simulink model "ES005A_TmplMonr"  (R2013b)
settings: Solver=FixedStepDiscrete  SolverMode=SingleTasking  StartTime=0.0  StopTime=1  FixedStep=0.002  RelTol=1e-3
undefined symbols (not defined in the file): ELECGLBPRM_STRTUPSTDI_CNT_U08, ELECGLBPRM_STRTUPSTTMPLMONININTESTSTRT_CNT_U08, IninFlt, RtFlt, SpiConf_SpiChannel_TmplMonrCh1, SpiConf_SpiChannel_TmplMonrCh2, SpiConf_SpiChannel_TmplMonrCh3, SpiConf_SpiSequence_TmplMonrSeq1, SpiConf_SpiSequence_TmplMonrSeq2, SpiConf_SpiSequence_TmplMonrSeq3, STD_HIGH, STD_LOW, TMPLMONRCFGREG1READVAL_CNT_U16, TMPLMONRCFGREG1WRVAL_CNT_U16, TMPLMONRSTSREG2READVAL_CNT_U16, TMPLMONRWDGMODKEYWORD1_CNT_U16, TMPLMONRWDGMODKEYWORD2_CNT_U16, TMPLMONRWDGMODKEYWORD3_CNT_U16, TrigReg1
libraries: simulink x12
(part 1 of 4)
settings Model: Creator=HZY4G9  LastModifiedBy=fz41t8
settings SolverCC: AutoInsertRateTranBlk=on  InsertRTBMode=Always
settings DataIOCC: LimitDataPoints=off  SaveFormat=Structure  ReturnWorkspaceOutputs=on
settings OptimizationCC: BlockReduction=off  InlineParams=on  ZeroExternalMemoryAtStartup=off  ZeroInternalMemoryAtStartup=off  OptimizeModelRefInitCode=on  LifeSpan=1
settings DebuggingCC: SignalInfNanChecking=error  SignalRangeChecking=warning  UnderspecifiedInitializationDetection=Simplified  SolverPrmCheckMsg=error  InheritedTsInSrcMsg=error  DiscreteInheritContinuousMsg=error  SingleTaskRateTransMsg=error  TasksWithSamePriorityMsg=error  SigSpecEnsureSampleTimeMsg=error  CheckMatrixSingularityMsg=error  ParameterUnderflowMsg=error  ParameterPrecisionLossMsg=error  ParameterTunabilityLossMsg=error  FixptConstUnderflowMsg=warning  FixptConstOverflowMsg=warning  VectorMatrixConversionMsg=error  SignalLabelMismatchMsg=error  UnconnectedInputMsg=error  UnconnectedOutputMsg=error  UnconnectedLineMsg=error  SFcnCompatibilityMsg=error  UniqueDataStoreMsg=warning  BusObjectLabelMismatch=error  RootOutportRequireBusObject=error  AssertControl=DisableAll  ModelReferenceIOMsg=error  ModelReferenceVersionMismatchMessage=warning  ModelReferenceIOMismatchMessage=error  ModelReferenceCSMismatchMessage=warning  ModelReferenceDataLoggingMessage=error  StateNameClashWarn=warning  StrictBusMsg=ErrorOnBusTreatedAsVector  NonBusSignalsTreatedAsBus=error  SFUnexpectedBacktrackingDiag=error  SFInvalidInputDataAccessInChartInitDiag=error  SFNoUnconditionalDefaultTransitionDiag=error  SFTransitionOutsideNaturalParentDiag=error  SFUnconditionalTransitionShadowingDiag=error  SFUndirectedBroadcastEventsDiag=error
settings ModelReferenceCC: ModelReferenceNumInstancesAllowed=Single
settings RTWCC: SystemTargetFile=autosar.tlc  GenCodeOnly=on  TemplateMakefile=ert_default_tmf  Description=AUTOSAR  GenerateReport=on  ProcessScript=autosar_make_rtw_hook  LaunchReport=on
settings CodeAppCC: GenerateComments=off  IgnoreCustomStorageClasses=off  CustomSymbolStrType=$N$R$M  CustomSymbolStrBlkIO=$N$M  SimulinkBlockComments=off
settings STFCustomTargetCC: ParMdlRefBuildCompliant=on  CompOptLevelCompliant=on  IncludeMdlTerminateFcn=off  CombineOutputUpdateFcns=on  SuppressErrorStatus=on  ERTFirstTimeCompliant=on  ERTCustomFileBanners=on  SupportNonFinite=off  SupportComplex=off  SupportContinuousTime=off  SupportNonInlinedSFcns=off  MATLABClassNameForMDSCustomization=Simulink.SoftwareTarget.ERTCustomization  AutosarCompliant=on  GRTInterface=off  SystemTargetFile=autosar.tlc
settings ERTTargetCC: CodeReplacementLibrary=ANSI_C  ConcurrentExecutionCompliant=off  IncludeMdlTerminateFcn=off  SuppressErrorStatus=on  SupportNonFinite=off  SupportComplex=off  ModelStepFunctionPrototypeControlCompliant=off  CPPClassGenCompliant=off  AutosarCompliant=on  InlinedParameterPlacement=NonHierarchical  ERTCustomFileTemplate=example_file_process.tlc  EnableUserReplacementTypes=on

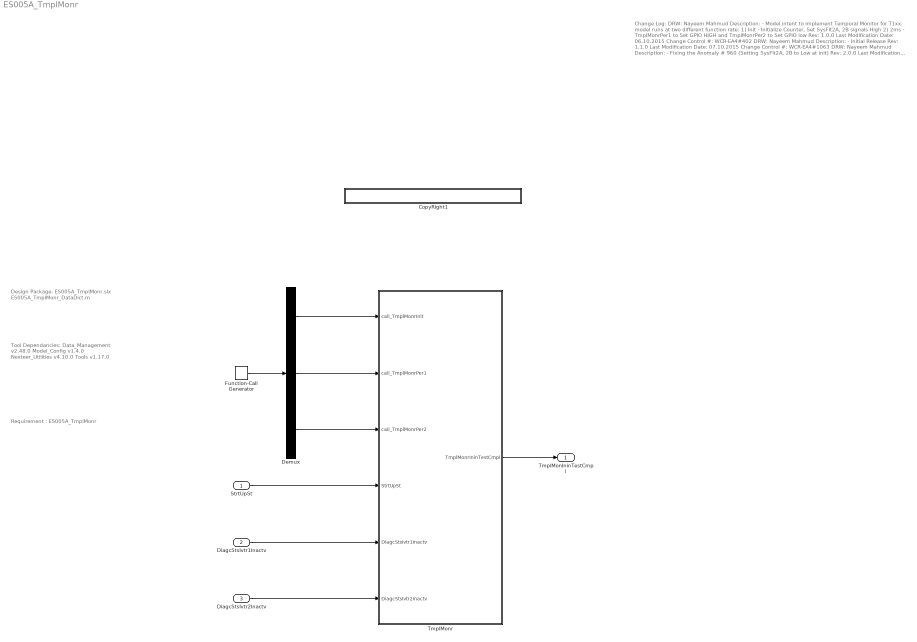
== system ES005A_TmplMonr ==
  note: Design Package:
      |
      | ES005A_TmplMonr.slx
      | ES005A_TmplMonr_DataDict.m
  note: Tool Dependancies:
      |
      | Data_Management v2.48.0
      | Model_Config v1.4.0
      | Nexteer_Utilities v4.10.0
      | Tools v1.17.0
  note: Requirement :
      | ES005A_TmplMonr
  note: Change Log:
      |
      | DRW: Nayeem Mahmud
      | Description:
      | - Model intent to implement Temporal Monitor for T1xx.
      |    model runs at two different function rate:
      |       1) Init - Initialize Counter, Set SysFlt2A, 2B signals High
      |       2) 2ms - TmplMonrPer1 to Set GPIO HIGH and TmplMonrPer2 to Set GPIO low
      |
      | Rev: 1.0.0
      | Last Modification Date: 06.10.2015
      | Change Control #: WCR-EA4#402
      | DRW: Nayeem Mahmud
      | Description:
      | - Initial Release
      |
      | Rev: 1.1.0
      | Last Modification Date: 07.10.2015
      | Change Control #: WCR-EA4#1063
      | DRW: Nayeem Mahmud
      | Description:
      | - Fixing the Anomaly # 960 (Setting SysFlt2A, 2B to Low at init)
      |
      | Rev: 2.0.0
      | Last Modification Date: 07.28.2015
      | Change Control #: WCR-EA4#773
      | DRW: Nayeem Mahmud
      | Description:
      | - Adding the start-up sequence
      |
      | Rev: 2.1.0
      | Last Modification Date: 08.3.2015
      | Change Control #: WCR-EA4#773
      | DRW: Nayeem Mahmud
      | Description:
      | - model and m file updates based on the review during code implementation (name mismatch, missing SetNtcSt, etc)
      |
      |
      | Rev: 2.2.0
      | Last Modification Date: 08.17.2015
      | Change Control #: WCR Anomaly#1338
      | DRW: Nayeem Mahmud
      | Description:
      | - Anomaly 1338 is fixed.
      |
      |
      | Rev: 2.3.0
      | Last Modification Date: 09.25.2015
      | Change Control #: WCR #
      | DRW: Nayeem Mahmud
      | Description:
      | - "SetNerrStDiOutp"  client funtion call has been replaced with "CtrlErrOut" with two arguments.
      | - NTC section has been added into the m file.
      |
      |
      | Rev: 2.4.0
      | Last Modification Date: 03.11.2016
      | Change Control #: Anomaly EA4#3982       Component CR EA4#4306       WCR # EA4#4372
      | DRW: Nayeem Mahmud
      | Description:
      | - Fixing the Anomaly # 3982 - Logic change in the if else condition to go between Init Test and RUN.
      |
      | Rev: 2.5.0
      | Last Modification Date: 06.13.2016
      | Change Control #: Anomaly EA4#5862      Component CR EA4#6197       WCR # EA4#6220
      | DRW: Jason Erlenbeck
      | Description:
      | - Fixing the Anomaly # 5862 - Only set NTC 0x040 after the retry event.
      |
      | Rev: 2.6.0
      | Last Modification Date: 08.11.2016
      | Change Control #: Component CR EA4#6710       WCR # EA4#6657
      | DRW: Raghavendran Mohan
      | Description:
      | - Adding a WD_Restart at the beginning of each warm init cycle.
      |
      | Rev: 2.7.0
      | Last Modification Date: 11.28.2016
      | Change Control #: Anomaly EA4#8519		Component CR EA4#8529       WCR # EA4#8531
      | DRW: Raghavendran Mohan
      | Description:
      | - Added DiagcStsIvtr1Inactv, DiagcStsIvtr2Inactv as inputs.
      | - Removed PowerOutputEnbale Feedback as input, removed physical input nError and removed physical output  POE.
      | - Added logic to set SysFlt2A and SysFlt2B
  StrtUpSt : Inport
  DiagcStsIvtr1Inactv : Inport  Port=2
  DiagcStsIvtr2Inactv : Inport  Port=3
  CopyRight1 : Subsystem  Description=|  mask(Copyright Information){none=on}
      | Copyright info block.                                               
      |                                                                     
      | Place copyright information at the top of every subsystem in design.
      mask prompts: none "No parameters"
      mask help: Place copyright information at the top of every subsystem in design.
      mask Display:
      | NxtrConf = 'Nexteer Confidential';
      | 
      | sys = bdroot; %handle for the current model ("system")
      | first = get_param(sys,'Created');
      | first = first(end-3:end);  %year is last four digits
      | 
      | last = get_param(sys,'LastModifiedDate');
      | if isempty(last)
      |     last = datestr(now,'yyyy');
      | else
      |     last = last(end-3:end);
      | end
      | 
      | if strcmp(first,last)
      |     fprintf('%s -- Copyright %s Nexteer',NxtrConf,first)
      | else
      |     fprintf('%s -- %s%s- %s Nexteer',NxtrConf,char(169),first,last)
      | end
  Demux : Demux  Outputs=3
  Function-Call Generator : simulink/Ports & Subsystems/Function-Call Generator  sample_time=.002  numberOfIterations=1
  TmplMonr : Subsystem  RequirementInfo={'linktype_rmi_doors' '0000c46a (/ESG Group/FDD Module Requirements/EA4 Specific/ES005A_TmplMonr)' '#ES005A_144' 'true' 'REQ: ES005A_144' '' } %GIDa_d95d113b_b32a_49cc_8d78_f5fb2b103391
  TmplMonIninTestCmpl : Outport
  wires:
  StrtUpSt/1 -> TmplMonr/4(StrtUpSt)
  TmplMonr/1(TmplMonrIninTestCmpl) -> TmplMonIninTestCmpl/1
  Demux/3 -> TmplMonr/3(call_TmplMonrPer2)
  Demux/2 -> TmplMonr/2(call_TmplMonrPer1)
  Demux/1 -> TmplMonr/1(call_TmplMonrInit)
  Function-Call Generator/1 -> Demux/1
  DiagcStsIvtr1Inactv/1 -> TmplMonr/5(DiagcStsIvtr1Inactv)
  DiagcStsIvtr2Inactv/1 -> TmplMonr/6(DiagcStsIvtr2Inactv)

== system ES005A_TmplMonr/CopyRight1 ==

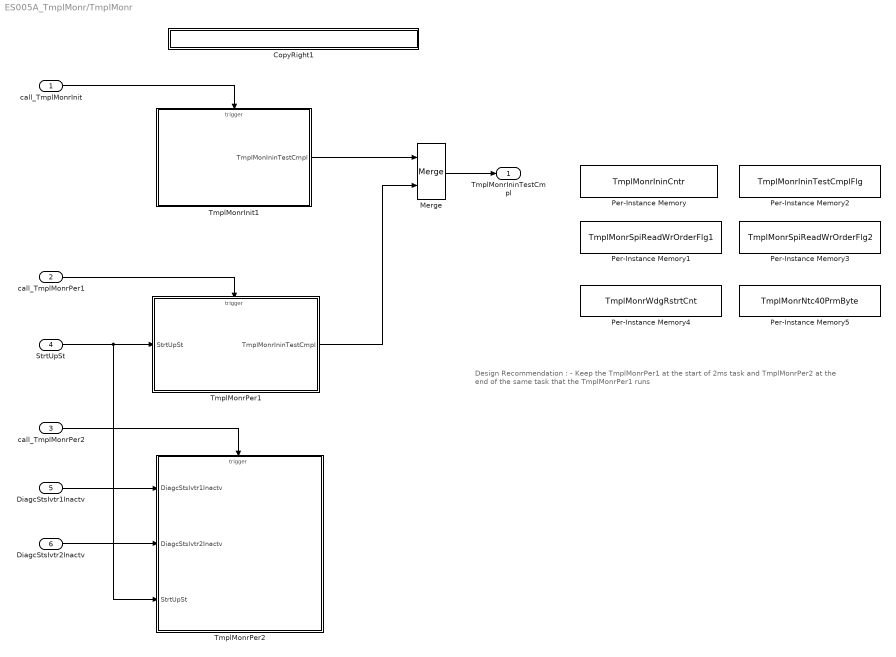
== system ES005A_TmplMonr/TmplMonr ==
  note: Design Recommendation :
      |
      | - Keep the TmplMonrPer1 at the start of 2ms task and TmplMonrPer2
      | at the end of the same task that the TmplMonrPer1 runs
  call_TmplMonrInit : Inport
  call_TmplMonrPer1 : Inport  Port=2
  call_TmplMonrPer2 : Inport  Port=3
  StrtUpSt : Inport  RequirementInfo={'linktype_rmi_doors' '0000c46a (/ESG Group/FDD Module Requirements/EA4 Specific/ES005A_TmplMonr)' '#ES005A_106' 'true' 'REQ: ES005A_106' '' } %GIDa_c29d43ec_8437_4b86_8b9f_d60d9d0f8c1f  Port=4
  DiagcStsIvtr1Inactv : Inport  Port=5
  DiagcStsIvtr2Inactv : Inport  Port=6
  CopyRight1 : Subsystem  Description=|  mask(Copyright Information){none=on}
      | Copyright info block.                                               
      |                                                                     
      | Place copyright information at the top of every subsystem in design.
      mask prompts: none "No parameters"
      mask help: Place copyright information at the top of every subsystem in design.
      mask Display:
      | NxtrConf = 'Nexteer Confidential';
      | 
      | sys = bdroot; %handle for the current model ("system")
      | first = get_param(sys,'Created');
      | first = first(end-3:end);  %year is last four digits
      | 
      | last = get_param(sys,'LastModifiedDate');
      | if isempty(last)
      |     last = datestr(now,'yyyy');
      | else
      |     last = last(end-3:end);
      | end
      | 
      | if strcmp(first,last)
      |     fprintf('%s -- Copyright %s Nexteer',NxtrConf,first)
      | else
      |     fprintf('%s -- %s%s- %s Nexteer',NxtrConf,char(169),first,last)
      | end
  Merge : Merge
  Per-Instance Memory : DataStoreMemory  RequirementInfo={'linktype_rmi_doors' '0000c46a (/ESG Group/FDD Module Requirements/EA4 Specific/ES005A_TmplMonr)' '#ES005A_169' 'true' 'REQ: ES005A_169' '' } %GIDa_d9f9d419_1585_49ea_bfa9_4f2c1d021cff  DataStoreName=TmplMonrIninCntr  StateMustResolveToSignalObject=on
  Per-Instance Memory1 : DataStoreMemory  DataStoreName=TmplMonrSpiReadWrOrderFlg1  StateMustResolveToSignalObject=on
  Per-Instance Memory2 : DataStoreMemory  DataStoreName=TmplMonrIninTestCmplFlg  OutDataTypeStr=boolean  StateMustResolveToSignalObject=on
  Per-Instance Memory3 : DataStoreMemory  DataStoreName=TmplMonrSpiReadWrOrderFlg2  StateMustResolveToSignalObject=on
  Per-Instance Memory4 : DataStoreMemory  DataStoreName=TmplMonrWdgRstrtCnt  StateMustResolveToSignalObject=on
  Per-Instance Memory5 : DataStoreMemory  DataStoreName=TmplMonrNtc40PrmByte  StateMustResolveToSignalObject=on
  TmplMonrInit1 : Subsystem
  TmplMonrPer1 : Subsystem  RequirementInfo={'linktype_rmi_doors' '0000c46a (/ESG Group/FDD Module Requirements/EA4 Specific/ES005A_TmplMonr)' '#ES005A_29' 'true' 'REQ: ES005A_29' '' ; 'linktype_rmi_doors' '0000c46a (/ESG Group/FDD Module Requirements/EA4 Specific/ES005A_TmplMonr)' '#ES005A_104' 'true' 'REQ: ES005A_104' '' } %GIDa_21503067_1abd_4975_a083_ff275a15b7aa
  TmplMonrPer2 : Subsystem  RequirementInfo={'linktype_rmi_doors' '0000c46a (/ESG Group/FDD Module Requirements/EA4 Specific/ES005A_TmplMonr)' '#ES005A_29' 'true' 'REQ: ES005A_29' '' ; 'linktype_rmi_doors' '0000c46a (/ESG Group/FDD Module Requirements/EA4 Specific/ES005A_TmplMonr)' '#ES005A_104' 'true' 'REQ: ES005A_104' '' } %GIDa_9e648429_fb1e_481f_a310_daf93cb17ebb
  TmplMonrIninTestCmpl : Outport  RequirementInfo={'linktype_rmi_doors' '0000c46a (/ESG Group/FDD Module Requirements/EA4 Specific/ES005A_TmplMonr)' '#ES005A_97' 'true' 'REQ: ES005A_97' '' } %GIDa_608f65af_4453_4e46_9bfc_731f93fa211f
  wires:
  call_TmplMonrInit/1 -> TmplMonrInit1/Trigger
  TmplMonrInit1/1(TmplMonIninTestCmpl) -> Merge/1
  call_TmplMonrPer1/1 -> TmplMonrPer1/Trigger
  call_TmplMonrPer2/1 -> TmplMonrPer2/Trigger
  TmplMonrPer1/1(TmplMonrIninTestCmpl) -> Merge/2
  StrtUpSt/1 -> TmplMonrPer2/3(StrtUpSt), TmplMonrPer1/1(StrtUpSt)
  Merge/1 -> TmplMonrIninTestCmpl/1
  DiagcStsIvtr2Inactv/1 -> TmplMonrPer2/2(DiagcStsIvtr2Inactv)
  DiagcStsIvtr1Inactv/1 -> TmplMonrPer2/1(DiagcStsIvtr1Inactv)

== system ES005A_TmplMonr/TmplMonr/CopyRight1 ==

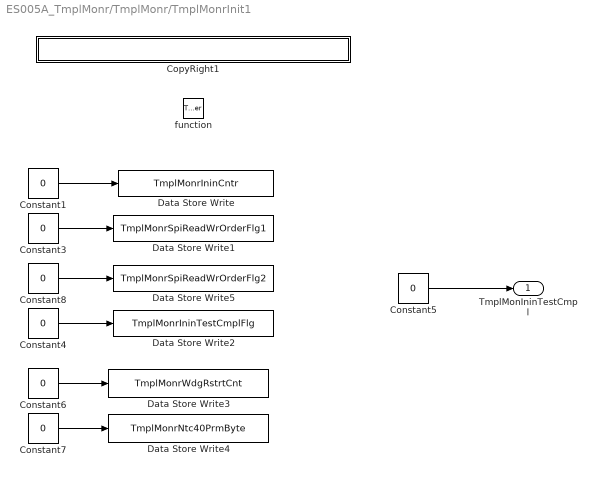
== system ES005A_TmplMonr/TmplMonr/TmplMonrInit1 ==
  function : TriggerPort  TriggerType=function-call
  Constant1 : Constant  Value=0  OutDataTypeStr=uint8
  Constant{3..5,8} (4 alike) : Constant  Value=0  OutDataTypeStr=boolean
  Constant6 : Constant  Value=0  OutDataTypeStr=uint8
  Constant7 : Constant  Value=0  OutDataTypeStr=uint8
  CopyRight1 : Subsystem  Description=|  mask(Copyright Information){none=on}
      | Copyright info block.                                               
      |                                                                     
      | Place copyright information at the top of every subsystem in design.
      mask prompts: none "No parameters"
      mask help: Place copyright information at the top of every subsystem in design.
      mask Display:
      | NxtrConf = 'Nexteer Confidential';
      | 
      | sys = bdroot; %handle for the current model ("system")
      | first = get_param(sys,'Created');
      | first = first(end-3:end);  %year is last four digits
      | 
      | last = get_param(sys,'LastModifiedDate');
      | if isempty(last)
      |     last = datestr(now,'yyyy');
      | else
      |     last = last(end-3:end);
      | end
      | 
      | if strcmp(first,last)
      |     fprintf('%s -- Copyright %s Nexteer',NxtrConf,first)
      | else
      |     fprintf('%s -- %s%s- %s Nexteer',NxtrConf,char(169),first,last)
      | end
  Data Store Write : DataStoreWrite  DataStoreName=TmplMonrIninCntr
  Data Store Write1 : DataStoreWrite  DataStoreName=TmplMonrSpiReadWrOrderFlg1
  Data Store Write2 : DataStoreWrite  DataStoreName=TmplMonrIninTestCmplFlg  DataStoreElements=TmplMonrIninTestCmplFlg
  Data Store Write3 : DataStoreWrite  DataStoreName=TmplMonrWdgRstrtCnt
  Data Store Write4 : DataStoreWrite  DataStoreName=TmplMonrNtc40PrmByte
  Data Store Write5 : DataStoreWrite  DataStoreName=TmplMonrSpiReadWrOrderFlg2
  TmplMonIninTestCmpl : Outport
  wires:
  Constant1/1 -> Data Store Write/1
  Constant5/1 -> TmplMonIninTestCmpl/1
  Constant3/1 -> Data Store Write1/1
  Constant4/1 -> Data Store Write2/1
  Constant6/1 -> Data Store Write3/1
  Constant7/1 -> Data Store Write4/1
  Constant8/1 -> Data Store Write5/1

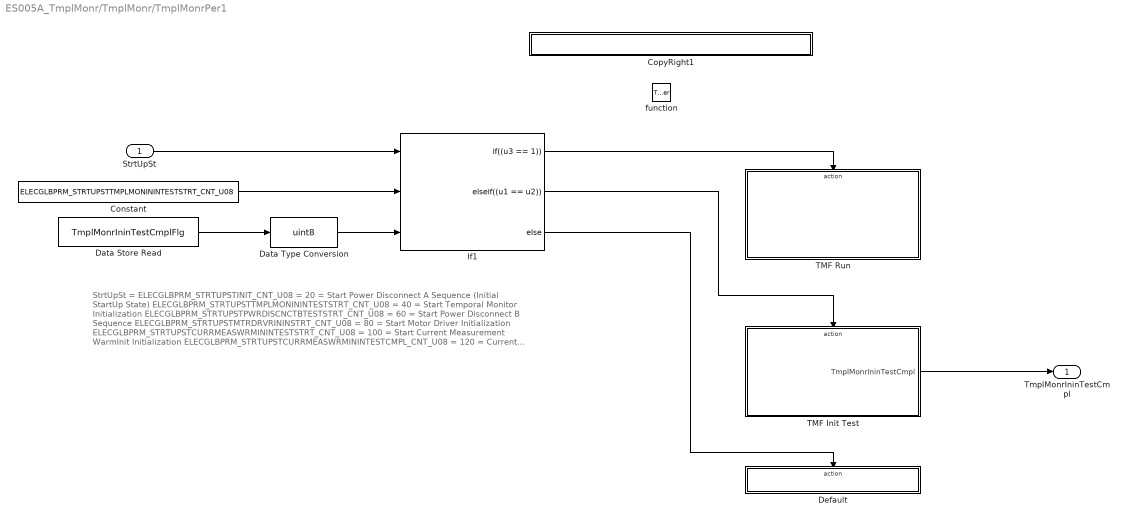
== system ES005A_TmplMonr/TmplMonr/TmplMonrPer1 ==
  note: StrtUpSt =
      | ELECGLBPRM_STRTUPSTINIT_CNT_U08                                               	=   20 	= Start Power Disconnect A Sequence (Initial StartUp State)
      | ELECGLBPRM_STRTUPSTTMPLMONININTESTSTRT_CNT_U08           	=   40 	= Start Temporal Monitor Initialization
      | ELECGLBPRM_STRTUPSTPWRDISCNCTBTESTSTRT_CNT_U08 		=   60 	= Start Power Disconnect B Sequence
      | ELECGLBPRM_STRTUPSTMTRDRVRININSTRT_CNT_U08 				=   80 	= Start Motor Driver Initialization
      | ELECGLBPRM_STRTUPSTCURRMEASWRMININTESTSTRT_CNT_U08 	= 100 	= Start Current Measurement WarmInit Initialization
      | ELECGLBPRM_STRTUPSTCURRMEASWRMININTESTCMPL_CNT_U08 	= 120 	= Current Measurement WarmInit Initialization Completed
      | ELECGLBPRM_STRTUPSTRUN_CNT_U08 							= 140 	= StartUp State in Run
      | ELECGLBPRM_STRTUPSTDI_CNT_U08 								= 160 	= StartUp State in Disable
  StrtUpSt : Inport  RequirementInfo={} %GIDa_e99920e6_f05f_4d7c_97e0_07210fe407a3
  function : TriggerPort  TriggerType=function-call
  Constant : Constant  Value=ELECGLBPRM_STRTUPSTTMPLMONININTESTSTRT_CNT_U08
  CopyRight1 : Subsystem  Description=|  mask(Copyright Information){none=on}
      | Copyright info block.                                               
      |                                                                     
      | Place copyright information at the top of every subsystem in design.
      mask prompts: none "No parameters"
      mask help: Place copyright information at the top of every subsystem in design.
      mask Display:
      | NxtrConf = 'Nexteer Confidential';
      | 
      | sys = bdroot; %handle for the current model ("system")
      | first = get_param(sys,'Created');
      | first = first(end-3:end);  %year is last four digits
      | 
      | last = get_param(sys,'LastModifiedDate');
      | if isempty(last)
      |     last = datestr(now,'yyyy');
      | else
      |     last = last(end-3:end);
      | end
      | 
      | if strcmp(first,last)
      |     fprintf('%s -- Copyright %s Nexteer',NxtrConf,first)
      | else
      |     fprintf('%s -- %s%s- %s Nexteer',NxtrConf,char(169),first,last)
      | end
  Data Store Read : DataStoreRead  DataStoreName=TmplMonrIninTestCmplFlg  DataStoreElements=TmplMonrIninTestCmplFlg
      settings: AttributesFormatString=%<Name>
  Data Type Conversion : DataTypeConversion  OutDataTypeStr=uint8
  Default : Subsystem  RequirementInfo={} %GIDa_701992d3_6d70_4ca5_b86b_b7f7e0f02188  TreatAsAtomicUnit=on
  If1 : If  RequirementInfo={'linktype_rmi_doors' '0000c46a (/ESG Group/FDD Module Requirements/EA4 Specific/ES005A_TmplMonr)' '#ES005A_108' 'true' 'REQ: ES005A_108' '' } %GIDa_2c5d92ce_735a_4987_a9b1_639812396b82  NumInputs=3  IfExpression=(u3 == 1)  ElseIfExpressions=(u1 == u2)
  TMF Init Test : Subsystem  RequirementInfo={'linktype_rmi_doors' '0000c46a (/ESG Group/FDD Module Requirements/EA4 Specific/ES005A_TmplMonr)' '#ES005A_32' 'true' 'REQ: ES005A_32' '' } %GIDa_2a4b0ef7_f795_469b_a72a_6f9ccacea2c5  TreatAsAtomicUnit=on
  TMF Run : Subsystem  RequirementInfo={'linktype_rmi_doors' '0000c46a (/ESG Group/FDD Module Requirements/EA4 Specific/ES005A_TmplMonr)' '#ES005A_168' 'true' 'REQ: ES005A_168' '' ; 'linktype_rmi_doors' '0000c46a (/ESG Group/FDD Module Requirements/EA4 Specific/ES005A_TmplMonr)' '#ES005A_125' 'true' 'REQ: ES005A_125' '' ; 'linktype_rmi_doors' '0000c46a (/ESG Group/FDD Module Requirements/EA4 Specific/ES005A_TmplMonr)' '#ES005A_124' 'true' 'REQ: ES005A_124' '' } %GIDa_7b07a290_cec0_4c21_ae9e_24b2761f4f96  TreatAsAtomicUnit=on
  TmplMonrIninTestCmpl : Outport  OutDataTypeStr=boolean
  wires:
  StrtUpSt/1 -> If1/1
  Constant/1 -> If1/2
  TMF Init Test/1(TmplMonrIninTestCmpl) -> TmplMonrIninTestCmpl/1
  Data Store Read/1 -> Data Type Conversion/1
  If1/3 -> Default/Action
  If1/1 -> TMF Run/Action
  If1/2 -> TMF Init Test/Action
  Data Type Conversion/1 -> If1/3

== system ES005A_TmplMonr/TmplMonr/TmplMonrPer2 ==
  note: SysFlt2A and Sysflt2B
  DiagcStsIvtr1Inactv : Inport
  DiagcStsIvtr2Inactv : Inport  Port=2
  StrtUpSt : Inport  RequirementInfo={'linktype_rmi_doors' '0000c46a (/ESG Group/FDD Module Requirements/EA4 Specific/ES005A_TmplMonr)' '#ES005A_106' 'true' 'REQ: ES005A_106' '' } %GIDa_d3b53d9b_e3bb_4cf5_b834_c5c47d08c4d5  Port=3
  function : TriggerPort  TriggerType=function-call
  Constant1 : Constant  Value=0  OutDataTypeStr=boolean
  CopyRight1 : Subsystem  Description=|  mask(Copyright Information){none=on}
      | Copyright info block.                                               
      |                                                                     
      | Place copyright information at the top of every subsystem in design.
      mask prompts: none "No parameters"
      mask help: Place copyright information at the top of every subsystem in design.
      mask Display:
      | NxtrConf = 'Nexteer Confidential';
      | 
      | sys = bdroot; %handle for the current model ("system")
      | first = get_param(sys,'Created');
      | first = first(end-3:end);  %year is last four digits
      | 
      | last = get_param(sys,'LastModifiedDate');
      | if isempty(last)
      |     last = datestr(now,'yyyy');
      | else
      |     last = last(end-3:end);
      | end
      | 
      | if strcmp(first,last)
      |     fprintf('%s -- Copyright %s Nexteer',NxtrConf,first)
      | else
      |     fprintf('%s -- %s%s- %s Nexteer',NxtrConf,char(169),first,last)
      | end
  IoHwAb_SetGpioTmplMonrWdg : Subsystem
  Subsystem : Subsystem
  wires:
  Constant1/1 -> IoHwAb_SetGpioTmplMonrWdg/1(PinSt)
  DiagcStsIvtr1Inactv/1 -> Subsystem/2(DiagcStsIvtr1Inactv)
  DiagcStsIvtr2Inactv/1 -> Subsystem/3(DiagcStsIvtr2Inactv)
  StrtUpSt/1 -> Subsystem/1(StrtUpSt)

== system ES005A_TmplMonr/TmplMonr/TmplMonrInit1/CopyRight1 ==

== system ES005A_TmplMonr/TmplMonr/TmplMonrPer1/CopyRight1 ==

== system ES005A_TmplMonr/TmplMonr/TmplMonrPer1/Default ==
  note: DO NOTHING
  Action Port : ActionPort  ActionType=else
  CopyRight1 : Subsystem  Description=|  mask(Copyright Information){none=on}
      | Copyright info block.                                               
      |                                                                     
      | Place copyright information at the top of every subsystem in design.
      mask prompts: none "No parameters"
      mask help: Place copyright information at the top of every subsystem in design.
      mask Display:
      | NxtrConf = 'Nexteer Confidential';
      | 
      | sys = bdroot; %handle for the current model ("system")
      | first = get_param(sys,'Created');
      | first = first(end-3:end);  %year is last four digits
      | 
      | last = get_param(sys,'LastModifiedDate');
      | if isempty(last)
      |     last = datestr(now,'yyyy');
      | else
      |     last = last(end-3:end);
      | end
      | 
      | if strcmp(first,last)
      |     fprintf('%s -- Copyright %s Nexteer',NxtrConf,first)
      | else
      |     fprintf('%s -- %s%s- %s Nexteer',NxtrConf,char(169),first,last)
      | end

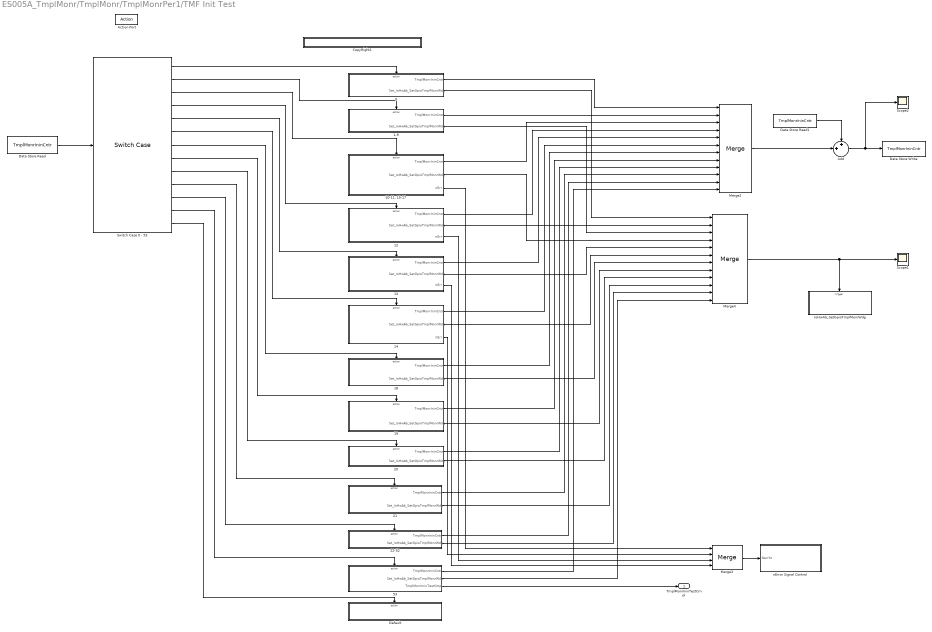
== system ES005A_TmplMonr/TmplMonr/TmplMonrPer1/TMF Init Test ==
  Action Port : ActionPort  ActionType=elseif
  0 : Subsystem  RequirementInfo={'linktype_rmi_doors' '0000c46a (/ESG Group/FDD Module Requirements/EA4 Specific/ES005A_TmplMonr)' '#ES005A_186' 'true' 'REQ: ES005A_186' '' } %GIDa_f709565a_7850_4a5e_bf12_c5c242c1cd69
  1-9 : Subsystem  RequirementInfo={'linktype_rmi_doors' '0000c46a (/ESG Group/FDD Module Requirements/EA4 Specific/ES005A_TmplMonr)' '#ES005A_107' 'true' 'REQ: ES005A_107' '' } %GIDa_f5138768_50b5_46d6_b020_8c73728c325c
  "10-11, 15-17" : Subsystem  RequirementInfo={'linktype_rmi_doors' '0000c46a (/ESG Group/FDD Module Requirements/EA4 Specific/ES005A_TmplMonr)' '#ES005A_107' 'true' 'REQ: ES005A_107' '' } %GIDa_6925605a_68a3_40d0_b458_ff3bce790b96
  12 : Subsystem  RequirementInfo={'linktype_rmi_doors' '0000c46a (/ESG Group/FDD Module Requirements/EA4 Specific/ES005A_TmplMonr)' '#ES005A_167' 'true' 'REQ: ES005A_167' '' ; 'linktype_rmi_doors' '0000c46a (/ESG Group/FDD Module Requirements/EA4 Specific/ES005A_TmplMonr)' '#ES005A_170' 'true' 'REQ: ES005A_170' '' } %GIDa_68f47203_75db_4fde_81b8_6da04bb37e60
  13 : Subsystem  RequirementInfo={'linktype_rmi_doors' '0000c46a (/ESG Group/FDD Module Requirements/EA4 Specific/ES005A_TmplMonr)' '#ES005A_167' 'true' 'REQ: ES005A_167' '' ; 'linktype_rmi_doors' '0000c46a (/ESG Group/FDD Module Requirements/EA4 Specific/ES005A_TmplMonr)' '#ES005A_170' 'true' 'REQ: ES005A_170' '' } %GIDa_fa4ceced_d8ba_4640_9bfa_b7203170527d
  14 : Subsystem  RequirementInfo={'linktype_rmi_doors' '0000c46a (/ESG Group/FDD Module Requirements/EA4 Specific/ES005A_TmplMonr)' '#ES005A_107' 'true' 'REQ: ES005A_107' '' } %GIDa_195c5f42_c7f7_445e_8ebf_65adf077b81b
  18 : Subsystem  RequirementInfo={'linktype_rmi_doors' '0000c46a (/ESG Group/FDD Module Requirements/EA4 Specific/ES005A_TmplMonr)' '#ES005A_170' 'true' 'REQ: ES005A_170' '' } %GIDa_626c2e42_567b_4ad3_8940_8fd5bf72a77a
  19 : Subsystem
  20 : Subsystem
  21 : Subsystem
  22-52 : Subsystem  RequirementInfo={'linktype_rmi_doors' '0000c46a (/ESG Group/FDD Module Requirements/EA4 Specific/ES005A_TmplMonr)' '#ES005A_168' 'true' 'REQ: ES005A_168' '' ; 'linktype_rmi_doors' '0000c46a (/ESG Group/FDD Module Requirements/EA4 Specific/ES005A_TmplMonr)' '#ES005A_124' 'true' 'REQ: ES005A_124' '' } %GIDa_802b0a81_9473_42e8_aae8_bc4a2fe5665f
  53 : Subsystem  RequirementInfo={'linktype_rmi_doors' '0000c46a (/ESG Group/FDD Module Requirements/EA4 Specific/ES005A_TmplMonr)' '#ES005A_168' 'true' 'REQ: ES005A_168' '' ; 'linktype_rmi_doors' '0000c46a (/ESG Group/FDD Module Requirements/EA4 Specific/ES005A_TmplMonr)' '#ES005A_124' 'true' 'REQ: ES005A_124' '' } %GIDa_61446ddd_207d_4cbd_8088_63e6ac5f381f
  Add : Sum  Inputs=++|
  CopyRight1 : Subsystem  Description=|  mask(Copyright Information){none=on}
      | Copyright info block.                                               
      |                                                                     
      | Place copyright information at the top of every subsystem in design.
      mask prompts: none "No parameters"
      mask help: Place copyright information at the top of every subsystem in design.
      mask Display:
      | NxtrConf = 'Nexteer Confidential';
      | 
      | sys = bdroot; %handle for the current model ("system")
      | first = get_param(sys,'Created');
      | first = first(end-3:end);  %year is last four digits
      | 
      | last = get_param(sys,'LastModifiedDate');
      | if isempty(last)
      |     last = datestr(now,'yyyy');
      | else
      |     last = last(end-3:end);
      | end
      | 
      | if strcmp(first,last)
      |     fprintf('%s -- Copyright %s Nexteer',NxtrConf,first)
      | else
      |     fprintf('%s -- %s%s- %s Nexteer',NxtrConf,char(169),first,last)
      | end
  Data Store Read : DataStoreRead  DataStoreName=TmplMonrIninCntr  DataStoreElements=TmplMonrIninCntr
  Data Store Read1 : DataStoreRead  DataStoreName=TmplMonrIninCntr
  Data Store Write : DataStoreWrite  DataStoreName=TmplMonrIninCntr
  Default : Subsystem
  IoHwAb_SetGpioTmplMonrWdg : Subsystem  RequirementInfo={'linktype_rmi_doors' '0000c46a (/ESG Group/FDD Module Requirements/EA4 Specific/ES005A_TmplMonr)' '#ES005A_104' 'true' 'REQ: ES005A_104' '' } %GIDa_16e4c81f_efba_49f3_a250_5a320869df18
  Merge2 : Merge  Inputs=12
  Merge3 : Merge  Inputs=4
  Merge4 : Merge  Inputs=12
  Scope1 : Scope
  Scope2 : Scope
  Switch Case 0 - 53 : SwitchCase  CaseConditions={[0],[1,2,3,4,5,6,7, 8,9], [10,11,15,16,17], [12], [13], [14], [18], [19], [20], [21], [22,23,24,25,26,27,28,29,30,31,32,33,34,35,36,37,38,39,40,41,42,43,44,45,46,47,48,49,50,51,52], [53]}
  nError Signal Control : Subsystem
  TmplMonrIninTestCmpl : Outport  OutDataTypeStr=boolean
  wires:
  Merge4/1 -> IoHwAb_SetGpioTmplMonrWdg/Trigger, Scope1/1
  Merge3/1 -> nError Signal Control/1(NerrSt)
  Add/1 -> Scope2/1, Data Store Write/1
  Data Store Read1/1 -> Add/1
  Merge2/1 -> Add/2
  Data Store Read/1 -> Switch Case 0 - 53/1
  Switch Case 0 - 53/2 -> 1-9/Action
  Switch Case 0 - 53/6 -> 14/Action
  Switch Case 0 - 53/4 -> 12/Action
  Switch Case 0 - 53/5 -> 13/Action
  Switch Case 0 - 53/7 -> 18/Action
  Switch Case 0 - 53/8 -> 19/Action
  Switch Case 0 - 53/9 -> 20/Action
  Switch Case 0 - 53/10 -> 21/Action
  Switch Case 0 - 53/11 -> 22-52/Action
  Switch Case 0 - 53/12 -> 53/Action
  Switch Case 0 - 53/13 -> Default/Action
  1-9/1(TmplMonrIninCntr) -> Merge2/2
  "10-11, 15-17"/1(TmplMonrIninCntr) -> Merge2/3
  12/1(TmplMonrIninCntr) -> Merge2/4
  13/1(TmplMonrIninCntr) -> Merge2/5
  18/1(TmplMonrIninCntr) -> Merge2/7
  19/1(TmplMonrIninCntr) -> Merge2/8
  20/1(TmplMonrIninCntr) -> Merge2/9
  21/1(TmplMonrIninCntr) -> Merge2/10
  22-52/1(TmplMonrIninCntr) -> Merge2/11
  53/1(TmplMonrIninCntr) -> Merge2/12
  1-9/2(Set_IoHwAb_SetGpioTmplMonrWdg) -> Merge4/3
  "10-11, 15-17"/2(Set_IoHwAb_SetGpioTmplMonrWdg) -> Merge4/4
  12/2(Set_IoHwAb_SetGpioTmplMonrWdg) -> Merge4/2
  13/2(Set_IoHwAb_SetGpioTmplMonrWdg) -> Merge4/5
  18/2(Set_IoHwAb_SetGpioTmplMonrWdg) -> Merge4/7
  19/2(Set_IoHwAb_SetGpioTmplMonrWdg) -> Merge4/8
  20/2(Set_IoHwAb_SetGpioTmplMonrWdg) -> Merge4/9
  21/2(Set_IoHwAb_SetGpioTmplMonrWdg) -> Merge4/10
  22-52/2(Set_IoHwAb_SetGpioTmplMonrWdg) -> Merge4/11
  53/2(Set_IoHwAb_SetGpioTmplMonrWdg) -> Merge4/12
  14/3(nErr) -> Merge3/2
  12/3(nErr) -> Merge3/3
  13/3(nErr) -> Merge3/4
  53/3(TmplMonrIninTestCmpl) -> TmplMonrIninTestCmpl/1
  Switch Case 0 - 53/3 -> "10-11, 15-17"/Action
  "10-11, 15-17"/3(nErr) -> Merge3/1
  14/1(TmplMonrIninCntr) -> Merge2/6
  14/2(Set_IoHwAb_SetGpioTmplMonrWdg) -> Merge4/6
  Switch Case 0 - 53/1 -> 0/Action
  0/1(TmplMonrIninCntr) -> Merge2/1
  0/2(Set_IoHwAb_SetGpioTmplMonrWdg) -> Merge4/1

== system ES005A_TmplMonr/TmplMonr/TmplMonrPer1/TMF Run ==
  Action Port : ActionPort  ActionType=then
  Constant1 : Constant  OutDataTypeStr=boolean
  CopyRight1 : Subsystem  Description=|  mask(Copyright Information){none=on}
      | Copyright info block.                                               
      |                                                                     
      | Place copyright information at the top of every subsystem in design.
      mask prompts: none "No parameters"
      mask help: Place copyright information at the top of every subsystem in design.
      mask Display:
      | NxtrConf = 'Nexteer Confidential';
      | 
      | sys = bdroot; %handle for the current model ("system")
      | first = get_param(sys,'Created');
      | first = first(end-3:end);  %year is last four digits
      | 
      | last = get_param(sys,'LastModifiedDate');
      | if isempty(last)
      |     last = datestr(now,'yyyy');
      | else
      |     last = last(end-3:end);
      | end
      | 
      | if strcmp(first,last)
      |     fprintf('%s -- Copyright %s Nexteer',NxtrConf,first)
      | else
      |     fprintf('%s -- %s%s- %s Nexteer',NxtrConf,char(169),first,last)
      | end
  Fault Condition - WD Run Fault : Subsystem  RequirementInfo={'linktype_rmi_doors' '0000c46a (/ESG Group/FDD Module Requirements/EA4 Specific/ES005A_TmplMonr)' '#ES005A_165' 'true' 'REQ: ES005A_165' '' } %GIDa_fa9bceb6_b2bb_4172_8dba_f786850c0fbe
  If1 : If  IfExpression=u1 == 1
  IoHwAb_GetGpioPwrOutpEnaFb : Subsystem
  IoHwAb_SetGpioTmplMonrWdg1 : Subsystem
  Normal Condition : Subsystem  RequirementInfo={'linktype_rmi_doors' '0000c46a (/ESG Group/FDD Module Requirements/EA4 Specific/ES005A_TmplMonr)' '#ES005A_166' 'true' 'REQ: ES005A_166' '' } %GIDa_0870c629_f590_4c25_b082_d0b0350c123f
  wires:
  Constant1/1 -> IoHwAb_SetGpioTmplMonrWdg1/1(PinSt)
  If1/1 -> Normal Condition/Action
  If1/2 -> Fault Condition - WD Run Fault/Action
  IoHwAb_GetGpioPwrOutpEnaFb/1(PinSt) -> If1/1

== system ES005A_TmplMonr/TmplMonr/TmplMonrPer2/CopyRight1 ==

== system ES005A_TmplMonr/TmplMonr/TmplMonrPer2/IoHwAb_SetGpioTmplMonrWdg ==
  PinSt : Inport
  Terminator : Terminator
  wires:
  PinSt/1 -> Terminator/1

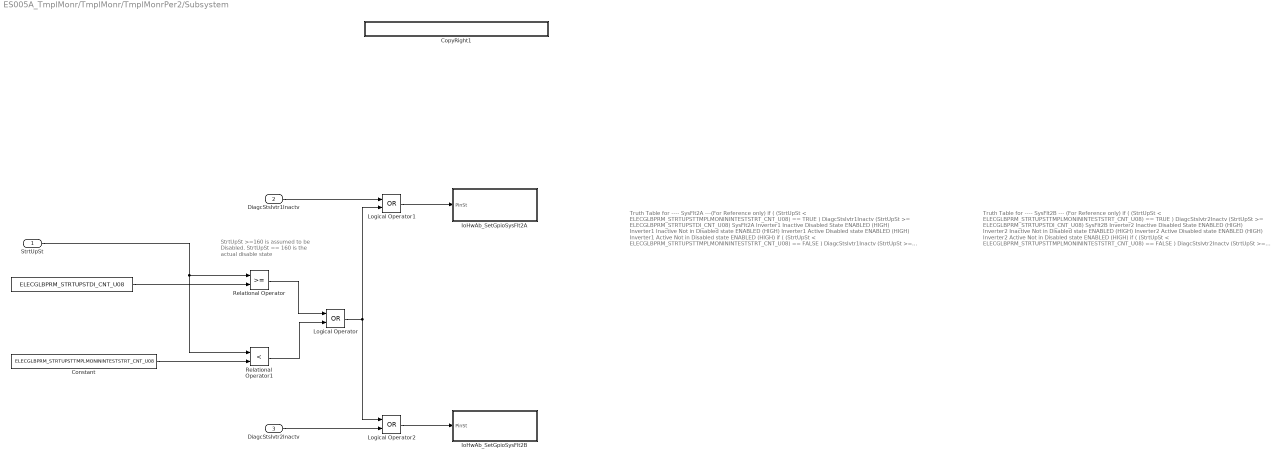
== system ES005A_TmplMonr/TmplMonr/TmplMonrPer2/Subsystem ==
  note: StrtUpSt >=160 is assumed
      | to be Disabled. StrtUpSt == 160
      | is the actual disable state
  note: Truth Table for 	----	SysFlt2A   ---(For Reference only)
      |
      |
      | if (	(StrtUpSt < ELECGLBPRM_STRTUPSTTMPLMONININTESTSTRT_CNT_U08)	==	TRUE	)
      |
      | DiagcStsIvtr1Inactv			(StrtUpSt >= ELECGLBPRM_STRTUPSTDI_CNT_U08)				SysFlt2A
      |
      | Inverter1 Inactive						Disabled State										ENABLED (HIGH)
      |
      | Inverter1 Inactive						Not in Disabled state									ENABLED (HIGH)
      |
      | Inverter1 Active						Disabled state										ENABLED (HIGH)
      |
      | Inverter1 Active						Not in Disabled state									ENABLED (HIGH)
      |
      |
      |
      | if (	(StrtUpSt < ELECGLBPRM_STRTUPSTTMPLMONININTESTSTRT_CNT_U08)	==	FALSE	)
      |
      | DiagcStsIvtr1Inactv			(StrtUpSt >= ELECGLBPRM_STRTUPSTDI_CNT_U08)				SysFlt2A
      |
      | Inverter1 Inactive						Disabled State										ENABLED (HIGH)
      |
      | Inverter1 Inactive						Not in Disabled state									ENABLED (HIGH)
      |
      | Inverter1 Active						Disabled state										ENABLED (HIGH)
      |
      | Inverter1 Active						Not in Disabled state									DISABLED (LOW)
  note: Truth Table for 	----	SysFlt2B   --- (For Reference only)
      |
      |
      | if (	(StrtUpSt < ELECGLBPRM_STRTUPSTTMPLMONININTESTSTRT_CNT_U08)	==	TRUE	)
      |
      | DiagcStsIvtr2Inactv			(StrtUpSt >= ELECGLBPRM_STRTUPSTDI_CNT_U08)				SysFlt2B
      |
      | Inverter2 Inactive						Disabled State										ENABLED (HIGH)
      |
      | Inverter2 Inactive						Not in Disabled state									ENABLED (HIGH)
      |
      | Inverter2 Active						Disabled state										ENABLED (HIGH)
      |
      | Inverter2 Active						Not in Disabled state									ENABLED (HIGH)
      |
      |
      |
      | if (	(StrtUpSt < ELECGLBPRM_STRTUPSTTMPLMONININTESTSTRT_CNT_U08)	==	FALSE	)
      |
      | DiagcStsIvtr2Inactv			(StrtUpSt >= ELECGLBPRM_STRTUPSTDI_CNT_U08)				SysFlt2B
      |
      | Inverter2 Inactive						Disabled State										ENABLED (HIGH)
      |
      | Inverter2 Inactive						Not in Disabled state									ENABLED (HIGH)
      |
      | Inverter2 Active						Disabled state										ENABLED (HIGH)
      |
      | Inverter2 Active						Not in Disabled state									DISABLED (LOW)
  StrtUpSt : Inport  RequirementInfo={'linktype_rmi_doors' '0000c46a (/ESG Group/FDD Module Requirements/EA4 Specific/ES005A_TmplMonr)' '#ES005A_106' 'true' 'REQ: ES005A_106' '' } %GIDa_2e1345e6_85c1_4fbf_9cb6_ca5d3d100667
  DiagcStsIvtr1Inactv : Inport  Port=2
  DiagcStsIvtr2Inactv : Inport  Port=3
  "   " : Constant  Value=ELECGLBPRM_STRTUPSTDI_CNT_U08
  Constant : Constant  Value=ELECGLBPRM_STRTUPSTTMPLMONININTESTSTRT_CNT_U08
  CopyRight1 : Subsystem  Description=|  mask(Copyright Information){none=on}
      | Copyright info block.                                               
      |                                                                     
      | Place copyright information at the top of every subsystem in design.
      mask prompts: none "No parameters"
      mask help: Place copyright information at the top of every subsystem in design.
      mask Display:
      | NxtrConf = 'Nexteer Confidential';
      | 
      | sys = bdroot; %handle for the current model ("system")
      | first = get_param(sys,'Created');
      | first = first(end-3:end);  %year is last four digits
      | 
      | last = get_param(sys,'LastModifiedDate');
      | if isempty(last)
      |     last = datestr(now,'yyyy');
      | else
      |     last = last(end-3:end);
      | end
      | 
      | if strcmp(first,last)
      |     fprintf('%s -- Copyright %s Nexteer',NxtrConf,first)
      | else
      |     fprintf('%s -- %s%s- %s Nexteer',NxtrConf,char(169),first,last)
      | end
  IoHwAb_SetGpioSysFlt2A : Subsystem  RequirementInfo={'linktype_rmi_doors' '0000c46a (/ESG Group/FDD Module Requirements/EA4 Specific/ES005A_TmplMonr)' '#ES005A_102' 'true' 'REQ: ES005A_102' '' ; 'linktype_rmi_doors' '0000c46a (/ESG Group/FDD Module Requirements/EA4 Specific/ES005A_TmplMonr)' '#ES005A_187' 'true' 'REQ: ES005A_187' '' } %GIDa_bb4ab7a6_6ae0_4578_87bc_9a60ea566083
  IoHwAb_SetGpioSysFlt2B : Subsystem  RequirementInfo={'linktype_rmi_doors' '0000c46a (/ESG Group/FDD Module Requirements/EA4 Specific/ES005A_TmplMonr)' '#ES005A_103' 'true' 'REQ: ES005A_103' '' ; 'linktype_rmi_doors' '0000c46a (/ESG Group/FDD Module Requirements/EA4 Specific/ES005A_TmplMonr)' '#ES005A_188' 'true' 'REQ: ES005A_188' '' } %GIDa_2487adce_083a_426d_b374_b711a2e89481
  Logical Operator : Logic  Operator=OR  AllPortsSameDT=off  OutDataTypeStr=boolean
  Logical Operator1 : Logic  Operator=OR  AllPortsSameDT=off  OutDataTypeStr=boolean
  Logical Operator2 : Logic  Operator=OR  AllPortsSameDT=off  OutDataTypeStr=boolean
  Relational Operator : RelationalOperator  OutDataTypeStr=boolean
  Relational Operator1 : RelationalOperator  Operator=<  OutDataTypeStr=boolean
  wires:
  Logical Operator1/1 -> IoHwAb_SetGpioSysFlt2A/1(PinSt)
  Logical Operator2/1 -> IoHwAb_SetGpioSysFlt2B/1(PinSt)
  StrtUpSt/1 -> Relational Operator/1, Relational Operator1/1
  Constant/1 -> Relational Operator1/2
  DiagcStsIvtr1Inactv/1 -> Logical Operator1/1
  Relational Operator/1 -> Logical Operator/1
  Relational Operator1/1 -> Logical Operator/2
  Logical Operator/1 -> Logical Operator1/2, Logical Operator2/1
  DiagcStsIvtr2Inactv/1 -> Logical Operator2/2
  "   "/1 -> Relational Operator/2

== system ES005A_TmplMonr/TmplMonr/TmplMonrPer1/Default/CopyRight1 ==

== system ES005A_TmplMonr/TmplMonr/TmplMonrPer1/TMF Init Test/0 ==
  note: WD RESTART:
      |
      |
      |
      |
      |
      |
      |
      |
      |
      |
      |
      |
      |
      |
      |
      |
      |
      |
      |
      |
      |
      |
      |    Note: Transmit the Watchdog Mode Key Words in above sequence.
  Action Port : ActionPort  ActionType=case
  Constant : Constant  Value=0  OutDataTypeStr=boolean
  Constant2 : Constant  OutDataTypeStr=uint8
  CopyRight1 : Subsystem  Description=|  mask(Copyright Information){none=on}
      | Copyright info block.                                               
      |                                                                     
      | Place copyright information at the top of every subsystem in design.
      mask prompts: none "No parameters"
      mask help: Place copyright information at the top of every subsystem in design.
      mask Display:
      | NxtrConf = 'Nexteer Confidential';
      | 
      | sys = bdroot; %handle for the current model ("system")
      | first = get_param(sys,'Created');
      | first = first(end-3:end);  %year is last four digits
      | 
      | last = get_param(sys,'LastModifiedDate');
      | if isempty(last)
      |     last = datestr(now,'yyyy');
      | else
      |     last = last(end-3:end);
      | end
      | 
      | if strcmp(first,last)
      |     fprintf('%s -- Copyright %s Nexteer',NxtrConf,first)
      | else
      |     fprintf('%s -- %s%s- %s Nexteer',NxtrConf,char(169),first,last)
      | end
  Watchdog Mode Key: Word1 : Subsystem
  Watchdog Mode Key: Word2 : Subsystem
  Watchdog Mode Key: Word3 : Subsystem
  TmplMonrIninCntr : Outport
  Set_IoHwAb_SetGpioTmplMonrWdg : Outport  Port=2
  wires:
  Constant/1 -> Set_IoHwAb_SetGpioTmplMonrWdg/1
  Constant2/1 -> TmplMonrIninCntr/1

== system ES005A_TmplMonr/TmplMonr/TmplMonrPer1/TMF Init Test/1-9 ==
  Action Port : ActionPort  ActionType=case
  Constant : Constant  OutDataTypeStr=boolean
  Constant2 : Constant  OutDataTypeStr=uint8
  CopyRight1 : Subsystem  Description=|  mask(Copyright Information){none=on}
      | Copyright info block.                                               
      |                                                                     
      | Place copyright information at the top of every subsystem in design.
      mask prompts: none "No parameters"
      mask help: Place copyright information at the top of every subsystem in design.
      mask Display:
      | NxtrConf = 'Nexteer Confidential';
      | 
      | sys = bdroot; %handle for the current model ("system")
      | first = get_param(sys,'Created');
      | first = first(end-3:end);  %year is last four digits
      | 
      | last = get_param(sys,'LastModifiedDate');
      | if isempty(last)
      |     last = datestr(now,'yyyy');
      | else
      |     last = last(end-3:end);
      | end
      | 
      | if strcmp(first,last)
      |     fprintf('%s -- Copyright %s Nexteer',NxtrConf,first)
      | else
      |     fprintf('%s -- %s%s- %s Nexteer',NxtrConf,char(169),first,last)
      | end
  TmplMonrIninCntr : Outport
  Set_IoHwAb_SetGpioTmplMonrWdg : Outport  Port=2
  wires:
  Constant2/1 -> TmplMonrIninCntr/1
  Constant/1 -> Set_IoHwAb_SetGpioTmplMonrWdg/1

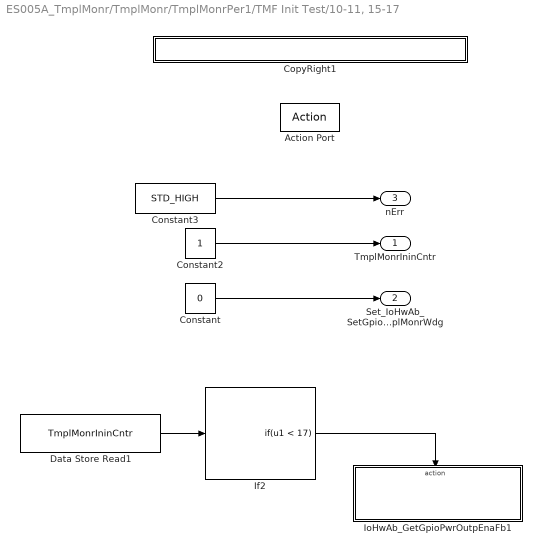
== system ES005A_TmplMonr/TmplMonr/TmplMonrPer1/TMF Init Test/10-11, 15-17 ==
  Action Port : ActionPort  ActionType=case
  Constant : Constant  Value=0  OutDataTypeStr=boolean
  Constant2 : Constant  OutDataTypeStr=uint8
  Constant3 : Constant  Value=STD_HIGH  OutDataTypeStr=uint8
  CopyRight1 : Subsystem  Description=|  mask(Copyright Information){none=on}
      | Copyright info block.                                               
      |                                                                     
      | Place copyright information at the top of every subsystem in design.
      mask prompts: none "No parameters"
      mask help: Place copyright information at the top of every subsystem in design.
      mask Display:
      | NxtrConf = 'Nexteer Confidential';
      | 
      | sys = bdroot; %handle for the current model ("system")
      | first = get_param(sys,'Created');
      | first = first(end-3:end);  %year is last four digits
      | 
      | last = get_param(sys,'LastModifiedDate');
      | if isempty(last)
      |     last = datestr(now,'yyyy');
      | else
      |     last = last(end-3:end);
      | end
      | 
      | if strcmp(first,last)
      |     fprintf('%s -- Copyright %s Nexteer',NxtrConf,first)
      | else
      |     fprintf('%s -- %s%s- %s Nexteer',NxtrConf,char(169),first,last)
      | end
  Data Store Read1 : DataStoreRead  DataStoreName=TmplMonrIninCntr
  If2 : If  RequirementInfo={'linktype_rmi_doors' '0000c46a (/ESG Group/FDD Module Requirements/EA4 Specific/ES005A_TmplMonr)' '#ES005A_163' 'true' 'REQ: ES005A_163' '' ; 'linktype_rmi_doors' '0000c46a (/ESG Group/FDD Module Requirements/EA4 Specific/ES005A_TmplMonr)' '#ES005A_172' 'true' 'REQ: ES005A_172' '' } %GIDa_befe16eb_941f_4fe1_a71f_516baf802abf  IfExpression=u1 < 17  ShowElse=off
  IoHwAb_GetGpioPwrOutpEnaFb1 : Subsystem
  TmplMonrIninCntr : Outport
  Set_IoHwAb_SetGpioTmplMonrWdg : Outport  Port=2
  nErr : Outport  Port=3
  wires:
  Constant2/1 -> TmplMonrIninCntr/1
  Constant/1 -> Set_IoHwAb_SetGpioTmplMonrWdg/1
  Constant3/1 -> nErr/1
  If2/1 -> IoHwAb_GetGpioPwrOutpEnaFb1/Action
  Data Store Read1/1 -> If2/1

== system ES005A_TmplMonr/TmplMonr/TmplMonrPer1/TMF Init Test/12 ==
  Action Port : ActionPort  ActionType=case
  Constant : Constant  Value=0  OutDataTypeStr=boolean
  Constant2 : Constant  OutDataTypeStr=uint8
  Constant3 : Constant  Value=STD_LOW  OutDataTypeStr=uint8
  CopyRight1 : Subsystem  Description=|  mask(Copyright Information){none=on}
      | Copyright info block.                                               
      |                                                                     
      | Place copyright information at the top of every subsystem in design.
      mask prompts: none "No parameters"
      mask help: Place copyright information at the top of every subsystem in design.
      mask Display:
      | NxtrConf = 'Nexteer Confidential';
      | 
      | sys = bdroot; %handle for the current model ("system")
      | first = get_param(sys,'Created');
      | first = first(end-3:end);  %year is last four digits
      | 
      | last = get_param(sys,'LastModifiedDate');
      | if isempty(last)
      |     last = datestr(now,'yyyy');
      | else
      |     last = last(end-3:end);
      | end
      | 
      | if strcmp(first,last)
      |     fprintf('%s -- Copyright %s Nexteer',NxtrConf,first)
      | else
      |     fprintf('%s -- %s%s- %s Nexteer',NxtrConf,char(169),first,last)
      | end
  TmplMonrIninCntr : Outport
  Set_IoHwAb_SetGpioTmplMonrWdg : Outport  Port=2
  nErr : Outport  Port=3
  wires:
  Constant/1 -> Set_IoHwAb_SetGpioTmplMonrWdg/1
  Constant2/1 -> TmplMonrIninCntr/1
  Constant3/1 -> nErr/1

== system ES005A_TmplMonr/TmplMonr/TmplMonrPer1/TMF Init Test/13 ==
  Action Port : ActionPort  ActionType=case
  Constant : Constant  Value=0  OutDataTypeStr=boolean
  Constant2 : Constant  OutDataTypeStr=uint8
  Constant3 : Constant  Value=STD_LOW  OutDataTypeStr=uint8
  CopyRight1 : Subsystem  Description=|  mask(Copyright Information){none=on}
      | Copyright info block.                                               
      |                                                                     
      | Place copyright information at the top of every subsystem in design.
      mask prompts: none "No parameters"
      mask help: Place copyright information at the top of every subsystem in design.
      mask Display:
      | NxtrConf = 'Nexteer Confidential';
      | 
      | sys = bdroot; %handle for the current model ("system")
      | first = get_param(sys,'Created');
      | first = first(end-3:end);  %year is last four digits
      | 
      | last = get_param(sys,'LastModifiedDate');
      | if isempty(last)
      |     last = datestr(now,'yyyy');
      | else
      |     last = last(end-3:end);
      | end
      | 
      | if strcmp(first,last)
      |     fprintf('%s -- Copyright %s Nexteer',NxtrConf,first)
      | else
      |     fprintf('%s -- %s%s- %s Nexteer',NxtrConf,char(169),first,last)
      | end
  Fault Condition - AND Gate : Subsystem  RequirementInfo={'linktype_rmi_doors' '0000c46a (/ESG Group/FDD Module Requirements/EA4 Specific/ES005A_TmplMonr)' '#ES005A_171' 'true' 'REQ: ES005A_171' '' } %GIDa_d3c588c6_6a5f_42e2_9afa_ebfca43d4f56
  If1 : If  RequirementInfo={'linktype_rmi_doors' '0000c46a (/ESG Group/FDD Module Requirements/EA4 Specific/ES005A_TmplMonr)' '#ES005A_171' 'true' 'REQ: ES005A_171' '' } %GIDa_e96b0668_38aa_4da5_867c_136a885774d5  IfExpression=u1 ~= 0  ShowElse=off
  IoHwAb_GetGpioPwrOutpEnaFb : Subsystem
  TmplMonrIninCntr : Outport
  Set_IoHwAb_SetGpioTmplMonrWdg : Outport  Port=2
  nErr : Outport  Port=3
  wires:
  If1/1 -> Fault Condition - AND Gate/Action
  Constant3/1 -> nErr/1
  Constant2/1 -> TmplMonrIninCntr/1
  IoHwAb_GetGpioPwrOutpEnaFb/1(PinSt) -> If1/1
  Constant/1 -> Set_IoHwAb_SetGpioTmplMonrWdg/1

== system ES005A_TmplMonr/TmplMonr/TmplMonrPer1/TMF Init Test/14 ==
  Action Port : ActionPort  ActionType=case
  Constant : Constant  Value=0  OutDataTypeStr=boolean
  Constant2 : Constant  OutDataTypeStr=uint8
  Constant3 : Constant  Value=STD_HIGH  OutDataTypeStr=uint8
  CopyRight1 : Subsystem  Description=|  mask(Copyright Information){none=on}
      | Copyright info block.                                               
      |                                                                     
      | Place copyright information at the top of every subsystem in design.
      mask prompts: none "No parameters"
      mask help: Place copyright information at the top of every subsystem in design.
      mask Display:
      | NxtrConf = 'Nexteer Confidential';
      | 
      | sys = bdroot; %handle for the current model ("system")
      | first = get_param(sys,'Created');
      | first = first(end-3:end);  %year is last four digits
      | 
      | last = get_param(sys,'LastModifiedDate');
      | if isempty(last)
      |     last = datestr(now,'yyyy');
      | else
      |     last = last(end-3:end);
      | end
      | 
      | if strcmp(first,last)
      |     fprintf('%s -- Copyright %s Nexteer',NxtrConf,first)
      | else
      |     fprintf('%s -- %s%s- %s Nexteer',NxtrConf,char(169),first,last)
      | end
  TmplMonrIninCntr : Outport
  Set_IoHwAb_SetGpioTmplMonrWdg : Outport  Port=2
  nErr : Outport  Port=3
  wires:
  Constant/1 -> Set_IoHwAb_SetGpioTmplMonrWdg/1
  Constant3/1 -> nErr/1
  Constant2/1 -> TmplMonrIninCntr/1

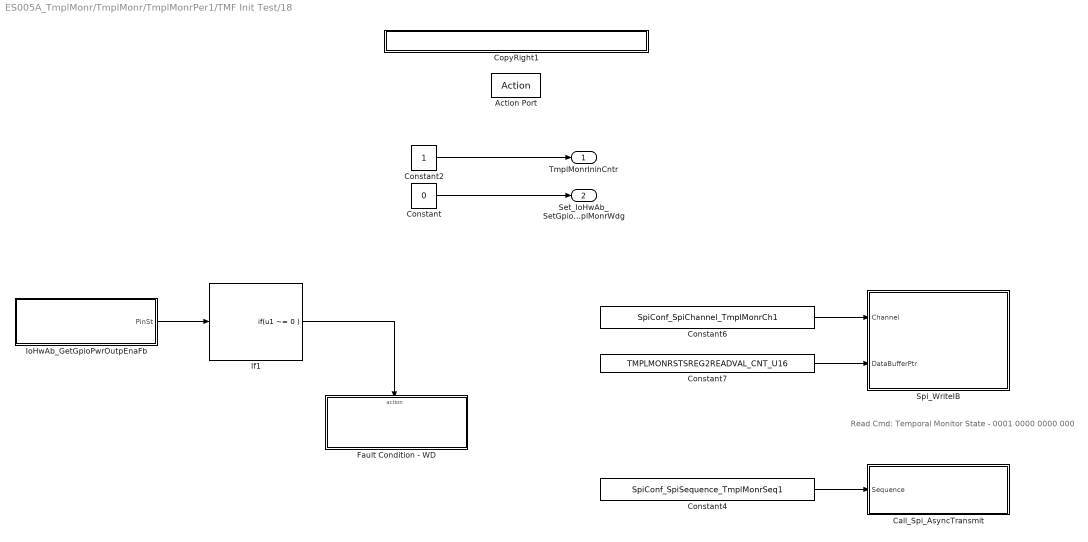
== system ES005A_TmplMonr/TmplMonr/TmplMonrPer1/TMF Init Test/18 ==
  note: Read Cmd: Temporal Monitor State - 0001 0000 0000 000
  Action Port : ActionPort  ActionType=case
  Call_Spi_AsyncTransmit : Subsystem
  Constant : Constant  Value=0  OutDataTypeStr=boolean
  Constant2 : Constant  OutDataTypeStr=uint8
  Constant4 : Constant  Value=SpiConf_SpiSequence_TmplMonrSeq1  OutDataTypeStr=uint8
  Constant6 : Constant  Value=SpiConf_SpiChannel_TmplMonrCh1  OutDataTypeStr=uint8
  Constant7 : Constant  Value=TMPLMONRSTSREG2READVAL_CNT_U16  OutDataTypeStr=uint16
  CopyRight1 : Subsystem  Description=|  mask(Copyright Information){none=on}
      | Copyright info block.                                               
      |                                                                     
      | Place copyright information at the top of every subsystem in design.
      mask prompts: none "No parameters"
      mask help: Place copyright information at the top of every subsystem in design.
      mask Display:
      | NxtrConf = 'Nexteer Confidential';
      | 
      | sys = bdroot; %handle for the current model ("system")
      | first = get_param(sys,'Created');
      | first = first(end-3:end);  %year is last four digits
      | 
      | last = get_param(sys,'LastModifiedDate');
      | if isempty(last)
      |     last = datestr(now,'yyyy');
      | else
      |     last = last(end-3:end);
      | end
      | 
      | if strcmp(first,last)
      |     fprintf('%s -- Copyright %s Nexteer',NxtrConf,first)
      | else
      |     fprintf('%s -- %s%s- %s Nexteer',NxtrConf,char(169),first,last)
      | end
  Fault Condition - WD : Subsystem  RequirementInfo={'linktype_rmi_doors' '0000c46a (/ESG Group/FDD Module Requirements/EA4 Specific/ES005A_TmplMonr)' '#ES005A_173' 'true' 'REQ: ES005A_173' '' } %GIDa_01ef8ac3_712e_44f4_a9ec_681d749c7a9c
  If1 : If  RequirementInfo={'linktype_rmi_doors' '0000c46a (/ESG Group/FDD Module Requirements/EA4 Specific/ES005A_TmplMonr)' '#ES005A_173' 'true' 'REQ: ES005A_173' '' } %GIDa_65f76126_3ff5_4264_8bb0_c66cd49af989  IfExpression=u1 ~= 0  ShowElse=off
  IoHwAb_GetGpioPwrOutpEnaFb : Subsystem
  Spi_WriteIB : Subsystem
  TmplMonrIninCntr : Outport
  Set_IoHwAb_SetGpioTmplMonrWdg : Outport  Port=2
  wires:
  Constant/1 -> Set_IoHwAb_SetGpioTmplMonrWdg/1
  Constant2/1 -> TmplMonrIninCntr/1
  IoHwAb_GetGpioPwrOutpEnaFb/1(PinSt) -> If1/1
  Constant4/1 -> Call_Spi_AsyncTransmit/1(Sequence)
  Constant6/1 -> Spi_WriteIB/1(Channel)
  Constant7/1 -> Spi_WriteIB/2(DataBufferPtr)
  If1/1 -> Fault Condition - WD/Action
